simulink model "MWP_OpenLoop"  (Simulink 10.0)
settings: Solver=ode5  StartTime=0  StopTime=100  FixedStep=Ts  RelTol=1e-3
values from neighbouring files (symbols this model uses):
  r0_init = 0    [Initial_Posture.m]
  rx_init = r_init(1)    [Initial_Posture.m]
  ry_init = r_init(2)    [Initial_Posture.m]
  rz_init = r_init(3)    [Initial_Posture.m]
  theta13_init = 0    [Initial_Posture.m]
  theta13d_init = 0    [Initial_Posture.m]
  theta23_init = 0    [Initial_Posture.m]
  theta23d_init = 0    [Initial_Posture.m]
  w3l_init = 0    [Initial_Posture.m]
  xCo_init = 0.5    [Initial_Posture.m]
  yCo_init = 0.5    [Initial_Posture.m]
  zCo_init = rw    [Initial_Posture.m]
settings Model: Creator=DanielleNasrallah  LastModifiedBy=kerrm
settings DataIOCC: SignalLoggingSaveFormat=ModelDataLogs  SignalLoggingName=sigsOut
settings OptimizationCC: ExpressionDepthLimit=2147483647  InitFltsAndDblsToZero=on
settings DebuggingCC: SaveWithParameterizedLinksMsg=none  SignalResolutionControl=TryResolveAllWithWarning  MultiTaskDSMMsg=warning  MultiTaskCondExecSysMsg=none  FcnCallInpInsideContextMsg=warning  StateNameClashWarn=warning
settings HardwareCC: TargetUnknown=on
settings GRTTargetCC: TargetFcnLib=ansi_tfl_tmw.mat  GeneratePreprocessorConditionals=Disable all
settings ConfigComp: CovExternalEMLEnable=off

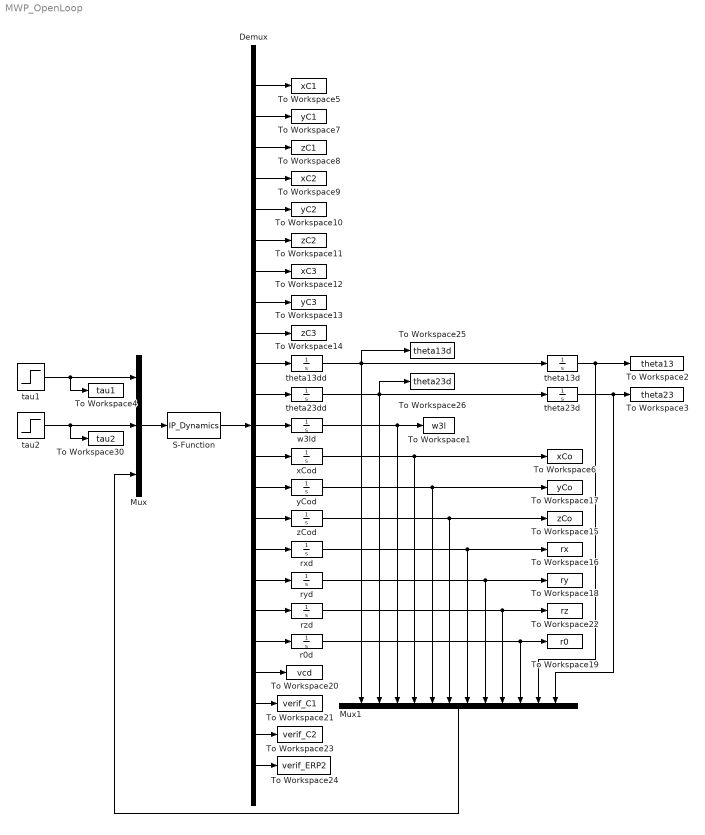
== system MWP_OpenLoop ==
  Demux : Demux  Outputs=23
  Mux : Mux  Inputs=3
  Mux1 : Mux  Inputs=12
  S-Function : S-Function  FunctionName=IP_Dynamics  SFunctionDeploymentMode=off  EnableBusSupport=off
  To Workspace1 : ToWorkspace  VariableName=w3l  SampleTime=-1
  To Workspace10 : ToWorkspace  VariableName=yC2  SampleTime=-1
  To Workspace11 : ToWorkspace  VariableName=zC2  SampleTime=-1
  To Workspace12 : ToWorkspace  VariableName=xC3  SampleTime=-1
  To Workspace13 : ToWorkspace  VariableName=yC3  SampleTime=-1
  To Workspace14 : ToWorkspace  VariableName=zC3  SampleTime=-1
  To Workspace15 : ToWorkspace  VariableName=zCo  SampleTime=-1
  To Workspace16 : ToWorkspace  VariableName=rx  SampleTime=-1
  To Workspace17 : ToWorkspace  VariableName=yCo  SampleTime=-1
  To Workspace18 : ToWorkspace  VariableName=ry  SampleTime=-1
  To Workspace19 : ToWorkspace  VariableName=r0  SampleTime=-1
  To Workspace2 : ToWorkspace  VariableName=theta13  SampleTime=-1
  To Workspace20 : ToWorkspace  VariableName=vcd  SampleTime=-1
  To Workspace21 : ToWorkspace  VariableName=verif_C1  SampleTime=-1
  To Workspace22 : ToWorkspace  VariableName=rz  SampleTime=-1
  To Workspace23 : ToWorkspace  VariableName=verif_C2  SampleTime=-1
  To Workspace24 : ToWorkspace  VariableName=verif_ERP2  SampleTime=-1
  To Workspace25 : ToWorkspace  VariableName=theta13d  SampleTime=-1
  To Workspace26 : ToWorkspace  VariableName=theta23d  SampleTime=-1
  To Workspace3 : ToWorkspace  VariableName=theta23  SampleTime=-1
  To Workspace30 : ToWorkspace  VariableName=tau2  SampleTime=-1
  To Workspace4 : ToWorkspace  VariableName=tau1  SampleTime=-1
  To Workspace5 : ToWorkspace  VariableName=xC1  SampleTime=-1
  To Workspace6 : ToWorkspace  VariableName=xCo  SampleTime=-1
  To Workspace7 : ToWorkspace  VariableName=yC1  SampleTime=-1
  To Workspace8 : ToWorkspace  VariableName=zC1  SampleTime=-1
  To Workspace9 : ToWorkspace  VariableName=xC2  SampleTime=-1
  r0d : Integrator  InitialCondition=r0_init
  rxd : Integrator  InitialCondition=rx_init
  ryd : Integrator  InitialCondition=ry_init
  rzd : Integrator  InitialCondition=rz_init
  tau1 : Step  Time=0  After=0.5  SampleTime=0
  tau2 : Step  Time=0  After=-0.5  SampleTime=0
  theta13d : Integrator  InitialCondition=theta13_init
  theta13dd : Integrator  InitialCondition=theta13d_init
  theta23d : Integrator  InitialCondition=theta23_init
  theta23dd : Integrator  InitialCondition=theta23d_init
  w3ld : Integrator  InitialCondition=w3l_init
  xCod : Integrator  InitialCondition=xCo_init
  yCod : Integrator  InitialCondition=yCo_init
  zCod : Integrator  InitialCondition=zCo_init
  wires:
  zCod/1 -> To Workspace15/1, Mux1/6
  Demux/1 -> To Workspace5/1
  Demux/2 -> To Workspace7/1
  Demux/3 -> To Workspace8/1
  Demux/4 -> To Workspace9/1
  Demux/5 -> To Workspace10/1
  Demux/6 -> To Workspace11/1
  Demux/7 -> To Workspace12/1
  Demux/8 -> To Workspace13/1
  Demux/9 -> To Workspace14/1
  theta13d/1 -> To Workspace2/1, Mux1/11
  theta13dd/1 -> Mux1/1, To Workspace25/1, theta13d/1
  theta23d/1 -> To Workspace3/1, Mux1/12
  theta23dd/1 -> theta23d/1, Mux1/2, To Workspace26/1
  w3ld/1 -> Mux1/3, To Workspace1/1
  r0d/1 -> To Workspace19/1, Mux1/10
  rzd/1 -> To Workspace22/1, Mux1/9
  xCod/1 -> To Workspace6/1, Mux1/4
  yCod/1 -> To Workspace17/1, Mux1/5
  rxd/1 -> To Workspace16/1, Mux1/7
  ryd/1 -> To Workspace18/1, Mux1/8
  Demux/10 -> theta13dd/1
  Demux/12 -> w3ld/1
  Demux/13 -> xCod/1
  Demux/14 -> yCod/1
  Demux/15 -> zCod/1
  Demux/16 -> rxd/1
  Demux/17 -> ryd/1
  Demux/19 -> r0d/1
  Demux/20 -> To Workspace20/1
  Demux/21 -> To Workspace21/1
  Demux/22 -> To Workspace23/1
  Demux/23 -> To Workspace24/1
  Demux/11 -> theta23dd/1
  Demux/18 -> rzd/1
  Mux1/1 -> Mux/3
  tau1/1 -> Mux/1, To Workspace4/1
  tau2/1 -> Mux/2, To Workspace30/1
  Mux/1 -> S-Function/1
  S-Function/1 -> Demux/1
